simulink model "pendulum2"  (R2021b)
settings: Solver=FixedStepAuto  StartTime=0.0  StopTime=100  FixedStep=0.01  RelTol=1e-3
libraries: cstblocks x1
settings Model: Creator=DELL  LastModifiedBy=DELL

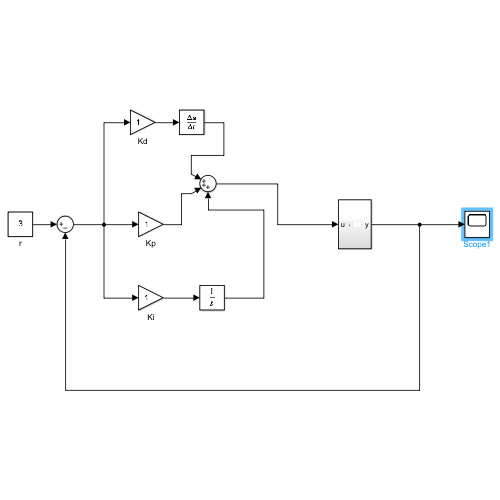
[thumbnail: Simulink's stored preview of the top-level diagram]
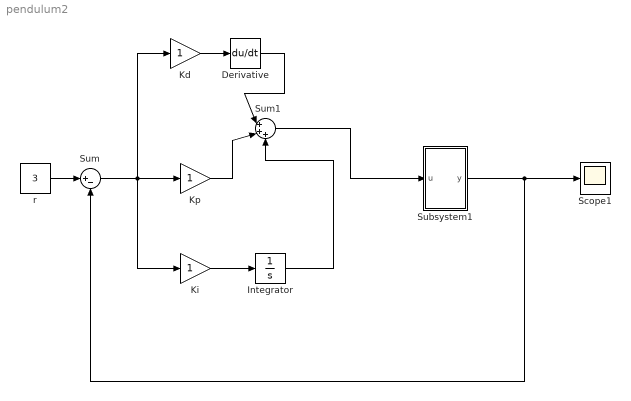
== system pendulum2 ==
  Derivative : Derivative
  Integrator : Integrator
  Kd : Gain
  Ki : Gain
  Kp : Gain
  Scope1 : Scope
  Subsystem1 : Subsystem
  Sum : Sum  Inputs=|+-
  Sum1 : Sum  Inputs=|+++
  r : Constant  Value=3
  wires:
  Subsystem1/1(y) -> Sum/2, Scope1/1
  Sum1/1 -> Subsystem1/1(u)
  r/1 -> Sum/1
  Sum/1 -> Kd/1, Ki/1, Kp/1
  Kp/1 -> Sum1/2
  Ki/1 -> Integrator/1
  Integrator/1 -> Sum1/3
  Kd/1 -> Derivative/1
  Derivative/1 -> Sum1/1

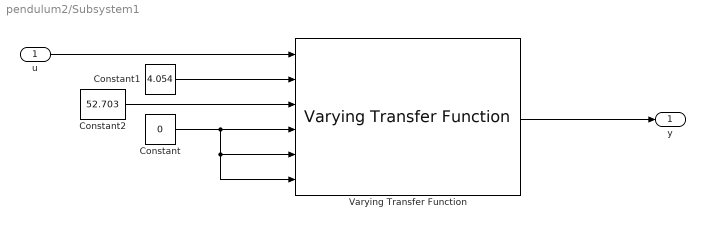
== system pendulum2/Subsystem1 ==
  u : Inport
  Constant : Constant  Value=0
  Constant1 : Constant  Value=4.054
  Constant2 : Constant  Value=52.703
  Varying Transfer Function : cstblocks/Linear Parameter Varying/Varying Transfer Function  N=2
  y : Outport
  wires:
  Varying Transfer Function/1 -> y/1
  Constant/1 -> Varying Transfer Function/6, Varying Transfer Function/5, Varying Transfer Function/4
  u/1 -> Varying Transfer Function/1
  Constant2/1 -> Varying Transfer Function/3
  Constant1/1 -> Varying Transfer Function/2
